simulink model "MRACDiretoTrab1Start"  (R2015a)
settings: Solver=ode45  StartTime=0.0  StopTime=360000  RelTol=1e-3
undefined symbols (not defined in the file): b, gamma, it, ref, theta_c_ini
libraries: simulink x4
settings Model: Creator=user  LastModifiedBy=user

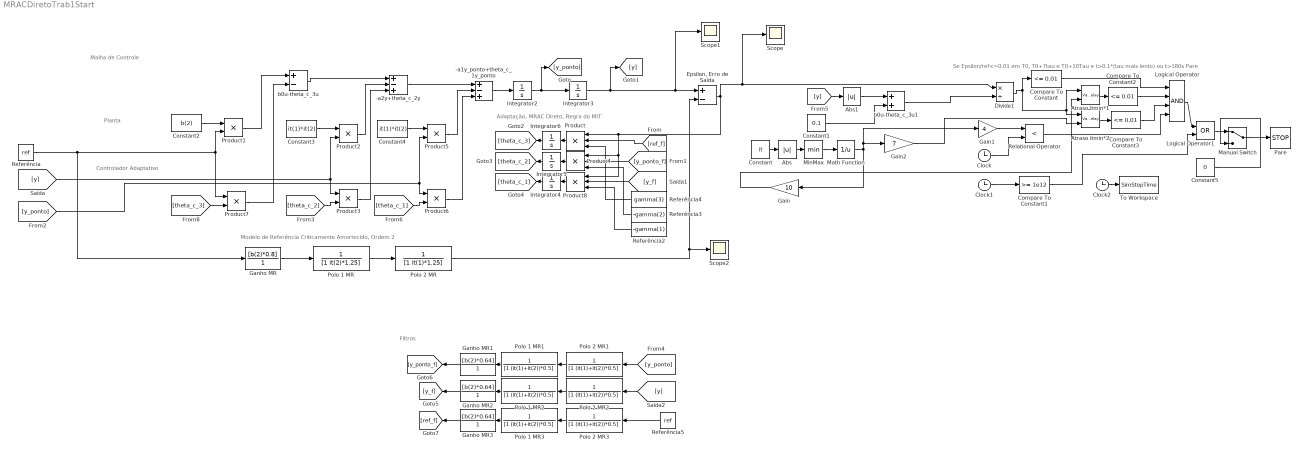
== system MRACDiretoTrab1Start ==
  note: Filtros
  note: Planta
  note: Malha de Controle
  note: Se Epsilon/ref<=0.01 em T0, T0+7tau e T0+10Tau e t>0.1*(tau mais lento) ou t>180s Pare
  note: Modelo de Referência Criticamente Amortecido, Ordem 2
  note: Controlador Adaptativo
  note: Adaptação, MRAC Direto, Regra do MIT
  "  Referência" : Constant  Value=ref
  "  Referência2" : Constant  Value=-gamma(1)
  "  Referência3" : Constant  Value=-gamma(2)
  "  Referência4" : Constant  Value=gamma(3)
  "  Referência5" : Constant  Value=ref
  -a1y_ponto+theta_c_1y_ponto : Sum  Inputs=+-+
  -a2y+theta_c_2y : Sum  Inputs=+-+
  Abs : Abs
  Abs1 : Abs
  Atraso itmin*1 : VariableTransportDelay  MaximumDelay=1000  MaximumPoints=65536
  Atraso itmin*2 : VariableTransportDelay  MaximumDelay=1000  MaximumPoints=65536
  Clock : Clock
  Clock1 : Clock
  Clock2 : Clock
  Compare To Constant : simulink/Logic and Bit Operations/Compare To Constant  relop=<=  const=0.01  OutDataTypeStr=boolean
  Compare To Constant1 : simulink/Logic and Bit Operations/Compare To Constant  relop=>=  const=1e12  OutDataTypeStr=boolean
  Compare To Constant2 : simulink/Logic and Bit Operations/Compare To Constant  relop=<=  const=0.01  OutDataTypeStr=boolean
  Compare To Constant3 : simulink/Logic and Bit Operations/Compare To Constant  relop=<=  const=0.01  OutDataTypeStr=boolean
  Constant : Constant  Value=it
  Constant1 : Constant  Value=0.1
  Constant2 : Constant  Value=b(2)
  Constant3 : Constant  Value=it(1)*it(2)
  Constant4 : Constant  Value=it(1)*it(2)
  Constant5 : Constant  Value=0
  Divide1 : Product  Inputs=*/
  "Epsilon, Erro de Saída" : Sum  Inputs=+-
  Gain : Gain  Gain=10
  Gain1 : Gain  Gain=4
  Gain2 : Gain  Gain=7
  Ganho MR : TransferFcn  Numerator=[b(2)*0.8]  Denominator=[1]
  Ganho MR1 : TransferFcn  Numerator=[b(2)*0.64]  Denominator=[1]
  Ganho MR2 : TransferFcn  Numerator=[b(2)*0.64]  Denominator=[1]
  Ganho MR3 : TransferFcn  Numerator=[b(2)*0.64]  Denominator=[1]
  Integrator2 : Integrator
  Integrator3 : Integrator
  Integrator4 : Integrator  InitialCondition=theta_c_ini(4)
  Integrator5 : Integrator  InitialCondition=theta_c_ini(3)
  Integrator6 : Integrator  InitialCondition=theta_c_ini(2)
  Logical Operator : Logic  Inputs=4  AllPortsSameDT=off  OutDataTypeStr=boolean
  Logical Operator1 : Logic  Operator=OR  AllPortsSameDT=off  OutDataTypeStr=boolean
  Manual Switch : ManualSwitch
  Math Function : Math  Operator=reciprocal  SaturateOnIntegerOverflow=on
  MinMax : MinMax
  Pare : Stop
  Polo 1 MR : TransferFcn  Denominator=[1 it(2)*1.25]
  Polo 1 MR1 : TransferFcn  Denominator=[1 (it(1)+it(2))*0.5]
  Polo 1 MR2 : TransferFcn  Denominator=[1 (it(1)+it(2))*0.5]
  Polo 1 MR3 : TransferFcn  Denominator=[1 (it(1)+it(2))*0.5]
  Polo 2 MR : TransferFcn  Denominator=[1 it(1)*1.25]
  Polo 2 MR1 : TransferFcn  Denominator=[1 (it(1)+it(2))*0.5]
  Polo 2 MR2 : TransferFcn  Denominator=[1 (it(1)+it(2))*0.5]
  Polo 2 MR3 : TransferFcn  Denominator=[1 (it(1)+it(2))*0.5]
  Product : Product  Inputs=3
  Product{1..3,5..7} (6 alike) : Product
  Product4 : Product  Inputs=3
  Product8 : Product  Inputs=3
  Relational Operator : RelationalOperator  Operator=<  OutDataTypeStr=boolean
  Scope : Scope
      settings: YMin=55.4  YMax=55.49
  Scope1 : Scope
      settings: YMin=51.1955  YMax=51.1995
  Scope2 : Scope
      settings: YMin=100  YMax=100  SaveName=ScopeData2
  To Workspace : ToWorkspace  VariableName=SimStopTime  SaveFormat=Timeseries  SampleTime=-1
  b0u-theta_c_3u : Sum  Inputs=+-
  b0u-theta_c_3u1 : Sum
  wires:
  "Epsilon, Erro de Saída"/1 -> Divide1/1, Scope/1, Product8/1, Product4/1, Product/1
  Ganho MR/1 -> Polo 1 MR/1
  Polo 1 MR/1 -> Polo 2 MR/1
  Polo 2 MR/1 -> Scope2/1, "Epsilon, Erro de Saída"/2
  Constant/1 -> Abs/1
  Abs/1 -> MinMax/1
  Gain/1 -> Atraso itmin*1/2
  Clock/1 -> Relational Operator/2
  Gain1/1 -> Relational Operator/1
  Compare To Constant/1 -> Logical Operator/1
  Divide1/1 -> Atraso itmin*1/1, Atraso itmin*2/1, Compare To Constant/1
  Relational Operator/1 -> Logical Operator/4
  Logical Operator/1 -> Logical Operator1/1
  Logical Operator1/1 -> Manual Switch/1
  Clock1/1 -> Compare To Constant1/1
  Compare To Constant1/1 -> Logical Operator1/2
  Clock2/1 -> To Workspace/1
  Integrator3/1 -> [y], Scope1/1, "Epsilon, Erro de Saída"/1
  Integrator2/1 -> [y_ponto], Integrator3/1
  -a1y_ponto+theta_c_1y_ponto/1 -> Integrator2/1
  -a2y+theta_c_2y/1 -> -a1y_ponto+theta_c_1y_ponto/1
  Product2/1 -> -a2y+theta_c_2y/2
  Constant3/1 -> Product2/1
  b0u-theta_c_3u/1 -> -a2y+theta_c_2y/1
  [y] -> Product2/2, Product3/1
  Product3/1 -> -a2y+theta_c_2y/3
  [theta_c_2] -> Product3/2
  Constant4/1 -> Product5/1
  [y_ponto] -> Product6/1, Product5/2
  [theta_c_1] -> Product6/2
  Product5/1 -> -a1y_ponto+theta_c_1y_ponto/2
  Product6/1 -> -a1y_ponto+theta_c_1y_ponto/3
  Constant2/1 -> Product1/1
  "  Referência"/1 -> Product1/2, Product7/1, Ganho MR/1
  [theta_c_3] -> Product7/2
  Product1/1 -> b0u-theta_c_3u/1
  Product7/1 -> b0u-theta_c_3u/2
  [ref_f] -> Product/2
  [y_ponto_f] -> Product4/2
  [y_f] -> Product8/2
  "  Referência4"/1 -> Product/3
  "  Referência3"/1 -> Product4/3
  "  Referência2"/1 -> Product8/3
  Polo 2 MR1/1 -> Polo 1 MR1/1
  Polo 1 MR1/1 -> Ganho MR1/1
  [y_ponto] -> Polo 2 MR1/1
  Polo 2 MR2/1 -> Polo 1 MR2/1
  Polo 1 MR2/1 -> Ganho MR2/1
  [y] -> Polo 2 MR2/1
  Ganho MR1/1 -> [y_ponto_f]
  Ganho MR2/1 -> [y_f]
  Polo 2 MR3/1 -> Polo 1 MR3/1
  Polo 1 MR3/1 -> Ganho MR3/1
  "  Referência5"/1 -> Polo 2 MR3/1
  Ganho MR3/1 -> [ref_f]
  Product8/1 -> Integrator4/1
  Integrator4/1 -> [theta_c_1]
  Product/1 -> Integrator6/1
  Integrator6/1 -> [theta_c_3]
  Product4/1 -> Integrator5/1
  Integrator5/1 -> [theta_c_2]
  Gain2/1 -> Atraso itmin*2/2
  Compare To Constant3/1 -> Logical Operator/3
  Compare To Constant2/1 -> Logical Operator/2
  Atraso itmin*1/1 -> Compare To Constant2/1
  Atraso itmin*2/1 -> Compare To Constant3/1
  Manual Switch/1 -> Pare/1
  Constant5/1 -> Manual Switch/2
  MinMax/1 -> Math Function/1
  Math Function/1 -> Gain1/1, Gain2/1, Gain/1
  Constant1/1 -> b0u-theta_c_3u1/2
  b0u-theta_c_3u1/1 -> Divide1/2
  [y] -> Abs1/1
  Abs1/1 -> b0u-theta_c_3u1/1
